simulink model "ld1_simulink"  (R2017b)
settings: Solver=VariableStepAuto  StartTime=0.0  StopTime=0.1  RelTol=1e-3
values from neighbouring files (symbols this model uses):
  Fs = 8000    [ld1.m]
  tau = 1e-3    (= 0.001)    [ld1.m]
undefined symbols (not defined in the file or in its folder): kcmpnd
libraries: simulink x1
settings Model: Creator=imants  LastModifiedBy=imants

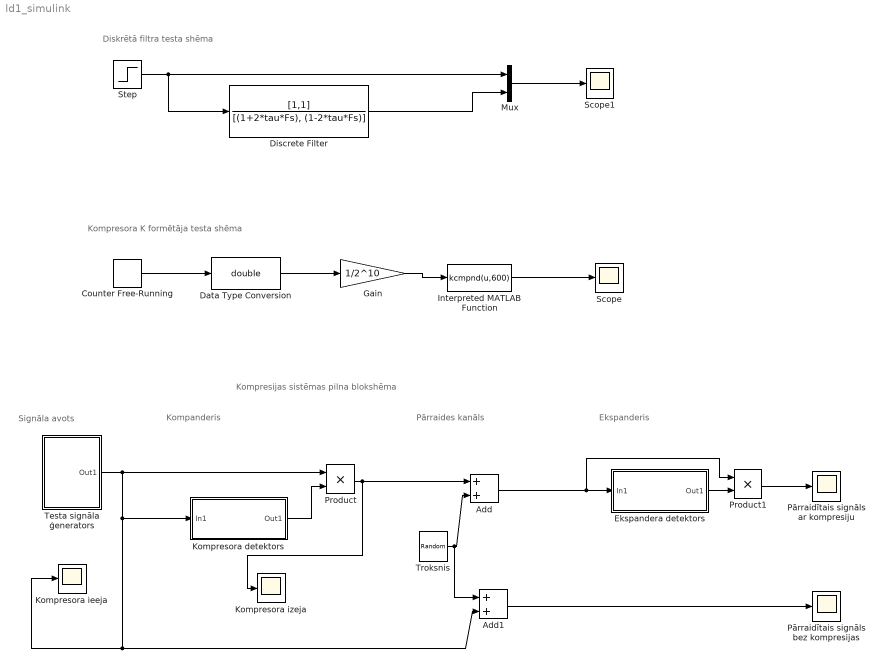
== system ld1_simulink ==
  note: Ekspanderis
  note: Pārraides kanāls
  note: Kompanderis
  note: Signāla avots
  note: Kompresijas sistēmas pilna blokshēma
  note: Kompresora K formētāja testa shēma
  note: Diskrētā filtra testa shēma
  Add : Sum
  Add1 : Sum
  Counter Free-Running : simulink/Sources/Counter Free-Running  NumBits=10  tsamp=1/Fs
  Data Type Conversion : DataTypeConversion  OutDataTypeStr=double
  Discrete Filter : DiscreteFilter  Numerator=[1,1]  Denominator=[(1+2*tau*Fs), (1-2*tau*Fs)]  FilterStructure=Direct form I  SampleTime=1/Fs
  Ekspandera detektors : Subsystem
  Gain : Gain  Gain=1/2^10
  Interpreted MATLAB Function : MATLABFcn  MATLABFcn=kcmpnd(u,600)  OutputDimensions=1
  "Kompresora ieeja " : Scope
  Kompresora izeja : Scope
  Kompresora detektors : Subsystem
  Mux : Mux  Inputs=2
  Product : Product
  Product1 : Product
  Pārraidītais signāls bez kompresijas : Scope
  Pārraidītais signāls ar kompresiju : Scope
  Scope : Scope
  Scope1 : Scope
  Step : Step  Before=1  After=0  SampleTime=1/Fs
  Testa signāla ģenerators : Subsystem
  Troksnis : UniformRandomNumber  Minimum=-0.1  Maximum=0.1  Seed=123  SampleTime=1/Fs
  wires:
  Discrete Filter/1 -> Mux/2
  Mux/1 -> Scope1/1
  Step/1 -> Discrete Filter/1, Mux/1
  Counter Free-Running/1 -> Data Type Conversion/1
  Data Type Conversion/1 -> Gain/1
  Gain/1 -> Interpreted MATLAB Function/1
  Interpreted MATLAB Function/1 -> Scope/1
  Testa signāla ģenerators/1(Out1) -> Product/1, Kompresora detektors/1(In1), Add1/2, "Kompresora ieeja "/1
  Kompresora detektors/1(Out1) -> Product/2
  Product/1 -> Add/1, Kompresora izeja/1
  Add1/1 -> Pārraidītais signāls bez kompresijas/1
  Troksnis/1 -> Add1/1, Add/2
  Add/1 -> Product1/1, Ekspandera detektors/1(In1)
  Ekspandera detektors/1(Out1) -> Product1/2
  Product1/1 -> Pārraidītais signāls ar kompresiju/1

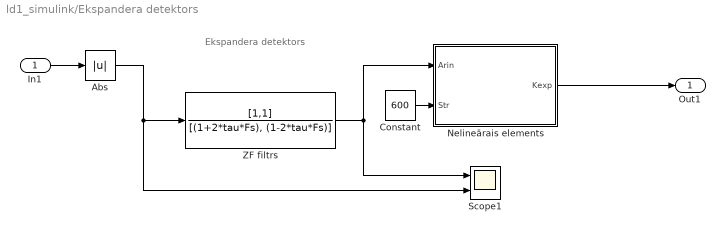
== system ld1_simulink/Ekspandera detektors ==
  note: Ekspandera detektors
  In1 : Inport
  Abs : Abs
  Constant : Constant  Value=600
  Nelineārais elements : MATLAB Function  TreatAsAtomicUnit=on
  Scope1 : Scope  NumInputPorts=2
  ZF filtrs : DiscreteFilter  Numerator=[1,1]  Denominator=[(1+2*tau*Fs), (1-2*tau*Fs)]  FilterStructure=Direct form I  SampleTime=1/Fs
  Out1 : Outport
  wires:
  In1/1 -> Abs/1
  Abs/1 -> Scope1/2, ZF filtrs/1
  Nelineārais elements/1(Kexp) -> Out1/1
  Constant/1 -> Nelineārais elements/2(Str)
  ZF filtrs/1 -> Nelineārais elements/1(Arin), Scope1/1

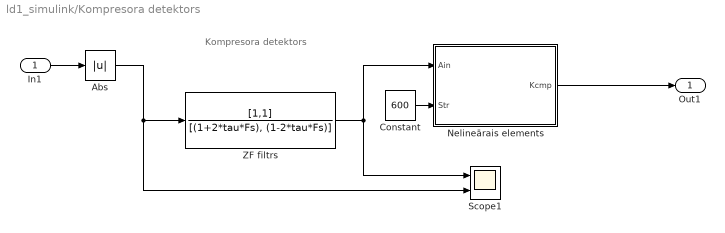
== system ld1_simulink/Kompresora detektors ==
  note: Kompresora detektors
  In1 : Inport
  Abs : Abs
  Constant : Constant  Value=600
  Nelineārais elements : MATLAB Function  TreatAsAtomicUnit=on
  Scope1 : Scope  NumInputPorts=2
  ZF filtrs : DiscreteFilter  Numerator=[1,1]  Denominator=[(1+2*tau*Fs), (1-2*tau*Fs)]  FilterStructure=Direct form I  SampleTime=1/Fs
  Out1 : Outport
  wires:
  In1/1 -> Abs/1
  Abs/1 -> Scope1/2, ZF filtrs/1
  Nelineārais elements/1(Kcmp) -> Out1/1
  Constant/1 -> Nelineārais elements/2(Str)
  ZF filtrs/1 -> Nelineārais elements/1(Ain), Scope1/1

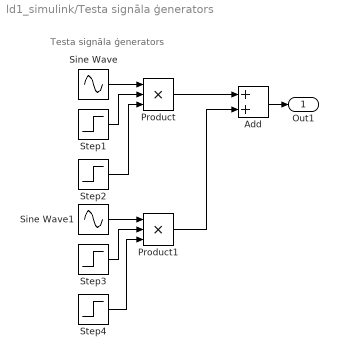
== system ld1_simulink/Testa signāla ģenerators ==
  note: Testa signāla ģenerators
  Add : Sum
  Product : Product  Inputs=3
  Product1 : Product  Inputs=3
  Sine Wave : Sin  Amplitude=0.7  Frequency=2*pi*Fs/10  SampleTime=0
  Sine Wave1 : Sin  Amplitude=0.3  Frequency=2*pi*Fs/10  SampleTime=0
  Step1 : Step  Time=0.005  SampleTime=1/Fs
  Step2 : Step  Time=0.03  Before=1  After=0  SampleTime=1/Fs
  Step3 : Step  Time=0.06  SampleTime=1/Fs
  Step4 : Step  Time=0.9  Before=1  After=0  SampleTime=1/Fs
  Out1 : Outport
  wires:
  Sine Wave/1 -> Product/1
  Product1/1 -> Add/2
  Product/1 -> Add/1
  Step4/1 -> Product1/3
  Add/1 -> Out1/1
  Step3/1 -> Product1/2
  Step2/1 -> Product/3
  Step1/1 -> Product/2
  Sine Wave1/1 -> Product1/1

== matlab function ld1_simulink/Ekspandera detektors/Nelineārais elements ==
  data: Arin input; Kexp output; Str input
function Kexp = kexpnd(Arin,Str)
% Kompresora pastiprinajuma koeficients
Kexp=zeros(size(Arin));
% Kexp=((Str + 1).^Arin - 1)./Str;
% Kexp = (exp(Arin.*log(Str+1)) - 1 ) ./ Str;
Kexp =  ((Str + 1).^Arin - 1)./(Arin.*Str);

== matlab function ld1_simulink/Kompresora detektors/Nelineārais elements ==
  data: Ain input; Kcmp output; Str input
function Kcmp = kcmpnd(Ain,Str)
% Kompresora pastiprinajuma koeficients
Kcmp=zeros(size(Ain));
Kcmp(Ain>0)=log10(Str*Ain(Ain>0)+1)./ ...
    Ain(Ain>0)/log10(Str+1);
Kcmp(Ain<=0) = Str/log(Str+1);
